simulink model "SIL_PIL_torque_extern"  (R2023b)
settings: Solver=VariableStepAuto  StartTime=0.0  StopTime=50  FixedStep=Ts  RelTol=1e-3  EnableMultiTasking=on
values from neighbouring files (symbols this model uses):
  k = kt    (= 1.45433391507)    [torque.m]
libraries: cstblocks x1
settings Model: SILPILSystemUnderTest=refmodels  CodeVerificationMode=processor-in-the-loop (pil)  ExtModeTrigDuration=10  Creator=giova  LastModifiedBy=giova
settings OptimizationCC: EnhancedBackFolding=on  PassReuseOutputArgsAs=Individual arguments  ZeroExternalMemoryAtStartup=off  ZeroInternalMemoryAtStartup=off  MaxStackSize=64  OptimizeBlockOrder=speed  DifferentSizesBufferReuse=on  OptimizationCustomize=off  EfficientTunableParamExpr=on
settings DebuggingCC: ParameterTunabilityLossMsg=error
settings HardwareCC: ProdBitPerPointer=32  ProdBitPerSizeT=32  ProdBitPerPtrDiffT=32  ProdLargestAtomicInteger=Long  ProdLargestAtomicFloat=Double  ProdWordSize=32  ProdLongLongMode=on  ProdHWDeviceType=ARM Compatible->ARM Cortex
settings SFSimCC: MATLABDynamicMemAlloc=off
settings RTWCC: Description=Embedded Coder  SystemTargetFile=ert.tlc  HardwareBoard=STM32 Nucleo F401RE  TemplateMakefile=ert_default_tmf  Toolchain=GNU Tools for ARM Embedded Processors  PortableWordSizes=on  CodeExecutionProfiling=on  CodeProfilingInstrumentation=coarse
settings CodeAppCC: ForceParamTrailComments=on  IgnoreCustomStorageClasses=off  OperatorAnnotations=on  SimulinkDataObjDesc=on  SFDataObjDesc=on  InsertBlockDesc=on
settings ERTTargetCC: ExtModeTransport=3  ExtModeStaticAlloc=on  ExtModeStaticAllocSize=2000  ExtModeMexFile=ext_xcp  ExtModeIntrfLevel=Level2 - Open

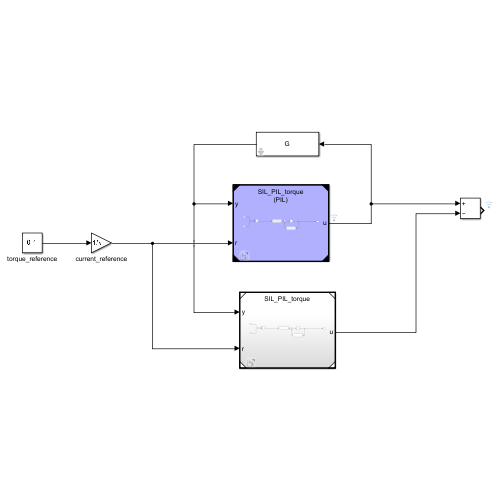
[thumbnail: Simulink's stored preview of the top-level diagram]
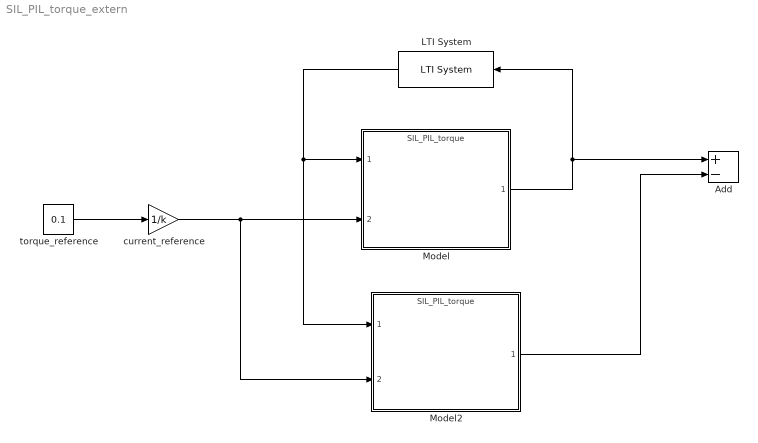
== system SIL_PIL_torque_extern ==
  Add : Sum  Inputs=+-
  LTI System : cstblocks/LTI System  sys=G  IC=[]  PadeOrder=0
  Model : ModelReference  ModelNameDialog=SIL_PIL_torque.slx  SimulationMode=Processor-in-the-loop (PIL)  ModelReferenceVersion=1.17
  Model2 : ModelReference  ModelNameDialog=SIL_PIL_torque.slx  SimulationMode=Normal  ModelReferenceVersion=1.17
  current_reference : Gain  Gain=1/k
  torque_reference : Constant  Value=0.1
  wires:
  torque_reference/1 -> current_reference/1
  LTI System/1 -> Model2/1, Model/1
  Model/1 -> LTI System/1, Add/1
  current_reference/1 -> Model2/2, Model/2
  Model2/1 -> Add/2
